simulink model "untitled"  (R2023b)
settings: Solver=VariableStepAuto  StartTime=0.0  StopTime=10  RelTol=1e-3
values from neighbouring files (symbols this model uses):
  A = [0 0 0 0 0 0 0 0 0 0 0 0 ... (16 elements, 4x4)]    [LMPC.mat]    (also in ball_balancing_platform.mat = [0 0 0 0 0 0 0 0 0 0 0 0 ... (64 elements, 8x8)]; new.mat = [0 0 0 0 0 0 0 0 0 0 0 0 ... (144 elements, 12x12)])
  B = [1 0 0 0 0 1 0 0 0 0 1 0 ... (16 elements, 4x4)]    [LMPC.mat]    (also in ball_balancing_platform.mat = [0 0 0 0 0 0 1 0 0 0 0 0 ... (16 elements, 8x2)]; new.mat = [0 0 0 0 0 0 0 0 0.769230769231 0 0 0 ... (48 elements, 12x4)
  C = [1 0 0 0 0 1 0 0 0 0 1 0 ... (16 elements, 4x4)]    [LMPC.mat]    (also in ball_balancing_platform.mat = [1 0 0 0 0 1 0 0 0 0 1 0 ... (32 elements, 4x8)]; new.mat = [1 0 0 0 0 0 0 1 0 0 0 0 ... (72 elements, 6x12)])
  D = [0 0 0 0 0 0 0 0 0 0 0 0 ... (16 elements, 4x4)]    [LMPC.mat]    (also in ball_balancing_platform.mat = [0  0; 0  0; 0  0; 0  0]; new.mat = [0 0 0 0 0 0 0 0 0 0 0 0 ... (24 elements, 6x4)])
libraries: mpclib x1, simulink x1, aerolibanimutils x1
settings Model: Creator=oem  LastModifiedBy=oem

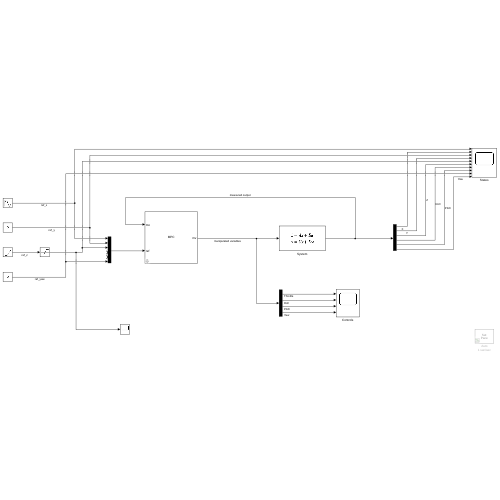
[thumbnail: Simulink's stored preview of the top-level diagram]
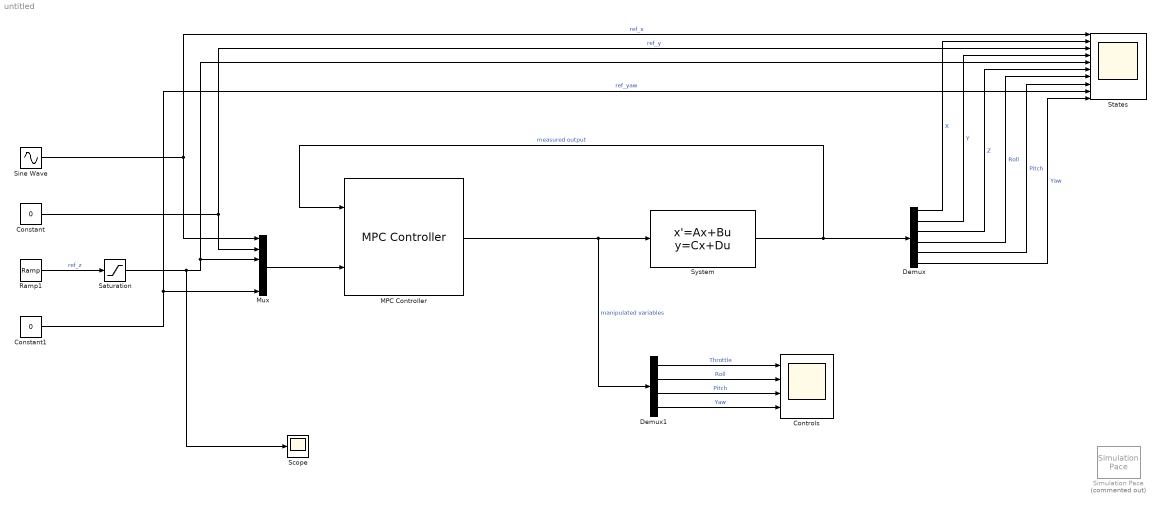
== system untitled ==
  Constant : Constant  Value=0
  Constant1 : Constant  Value=0
  Controls : Scope  NumInputPorts=4
  Demux : Demux  Outputs=6
  Demux1 : Demux
  MPC Controller : mpclib/MPC Controller  SCDEnableBlockLinearizationSpecification=on  mpcobj=mpc1  is_multiple=0  enable_value=0  return_u0=off  updateMPCinCallerWorkspace=on  md_inport=off  mv_inport=off  uref_inport=off  return_cost=off  return_mvseq=off  return_qpstatus=off  return_xseq=off  return_state=off  return_ovseq=off  state_inport=off  umin_inport=off  umax_inport=off  ymin_inport=off  ymax_inport=off  cc_inport=off  ywt_inport=off  uwt_inport=off  duwt_inport=off  rhoeps_inport=off  pm_inport=off  MaximumP=10  HorizonChoice=FixedHorizon  n_ts=0.1  n_p=10  n_mv=4  n_md=0  n_ud=0  n_mo=6  n_uo=0  BlockDataType=double  SampleTimeInherited=off  switch_inport=off
  Mux : Mux  Inputs=6
  Ramp1 : simulink/Sources/Ramp  slope=0.5  start=0  InitialOutput=0
  Saturation : Saturate  UpperLimit=1
  Scope : Scope
  Simulation Pace : aerolibanimutils/Simulation Pace  Commented=on  SimulationPace=1  SleepMode=Auto  OutputPaceError=off  SampleTime=1/30
  Sine Wave : Sin  Amplitude=4  SampleTime=0
  States : Scope  NumInputPorts=10
  System : StateSpace  A=A  B=B  C=C  D=D  InitialCondition=0
  wires:
  MPC Controller/1 -> Demux1/1, System/1  "manipulated variables"
  System/1 -> Demux/1, MPC Controller/1  "measured output"
  Mux/1 -> MPC Controller/2
  Sine Wave/1 -> States/1, Mux/1  "ref_x"
  Constant/1 -> States/3, Mux/2  "ref_y"
  Ramp1/1 -> Saturation/1  "ref_z"
  Constant1/1 -> States/9, Mux/6  "ref_yaw"
  Demux/1 -> States/2  "X"
  Demux/2 -> States/4  "Y"
  Demux/3 -> States/6  "Z"
  Demux/4 -> States/7  "Roll"
  Demux/5 -> States/8  "Pitch"
  Demux/6 -> States/10  "Yaw"
  Demux1/1 -> Controls/1  "Throttle"
  Demux1/2 -> Controls/2  "Roll"
  Demux1/4 -> Controls/4  "Yaw"
  Demux1/3 -> Controls/3  "Pitch"
  Saturation/1 -> Scope/1, States/5, Mux/3
